simulink model "quadtank_real_manual"  (Simulink 10.0)
settings: Solver=ode45  StartTime=0.0  StopTime=inf  RelTol=1e-3  EnableMultiTasking=on
libraries: simulink x2
settings Model: Creator=kristian  LastModifiedBy=olle
settings SolverCC: ZeroCrossAlgorithm=Non-adaptive
settings DataIOCC: LimitDataPoints=on  SignalLoggingSaveFormat=ModelDataLogs
settings OptimizationCC: ExpressionDepthLimit=2147483647  InitFltsAndDblsToZero=on
settings DebuggingCC: SolverPrmCheckMsg=warning  FcnCallInpInsideContextMsg=warning  StateNameClashWarn=warning
settings SFSimCC: SimUseLocalCustomCode=on  CustomCodeUndefinedFunction=FilterOut
settings RTWCC: RTWUseLocalCustomCode=on

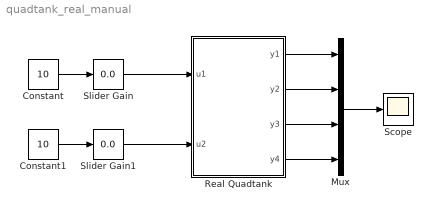
== system quadtank_real_manual ==
  Constant : Constant  Value=10
  Constant1 : Constant  Value=10
  Mux : Mux
  Real Quadtank : Subsystem  AncestorBlock=tank/Real Quadtank  VariantControl=Real  mask{h=0.05}
  Scope : Scope
  Slider Gain : simulink/Math Operations/Slider Gain  gain=0.0  low=0  high=1
  Slider Gain1 : simulink/Math Operations/Slider Gain  gain=0.0  low=0  high=1
  wires:
  Slider Gain/1 -> Real Quadtank/1(u1)
  Slider Gain1/1 -> Real Quadtank/2(u2)
  Constant/1 -> Slider Gain/1
  Constant1/1 -> Slider Gain1/1
  Mux/1 -> Scope/1
  Real Quadtank/1(y1) -> Mux/1
  Real Quadtank/2(y2) -> Mux/2
  Real Quadtank/3(y3) -> Mux/3
  Real Quadtank/4(y4) -> Mux/4

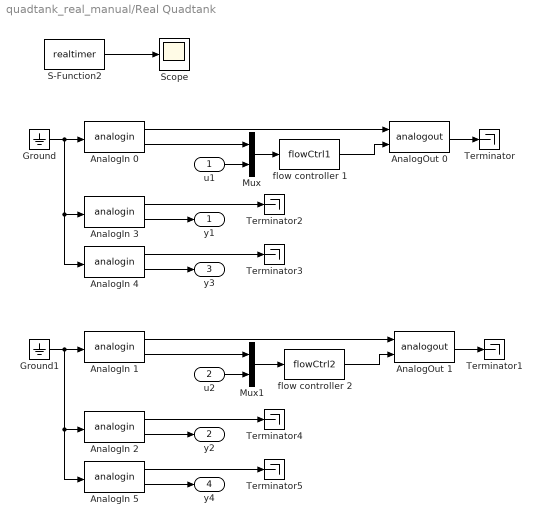
== system quadtank_real_manual/Real Quadtank ==
  u1 : Inport
  u2 : Inport  Port=2
  AnalogIn 0 : S-Function  FunctionName=analogin  Parameters=h [35]  SFunctionDeploymentMode=off  EnableBusSupport=off
  AnalogIn 1 : S-Function  FunctionName=analogin  Parameters=h [34]  SFunctionDeploymentMode=off  EnableBusSupport=off
  AnalogIn 2 : S-Function  FunctionName=analogin  Parameters=h [33]  SFunctionDeploymentMode=off  EnableBusSupport=off
  AnalogIn 3 : S-Function  FunctionName=analogin  Parameters=h [31]  SFunctionDeploymentMode=off  EnableBusSupport=off
  AnalogIn 4 : S-Function  FunctionName=analogin  Parameters=h [30]  SFunctionDeploymentMode=off  EnableBusSupport=off
  AnalogIn 5 : S-Function  FunctionName=analogin  Parameters=h [32]  SFunctionDeploymentMode=off  EnableBusSupport=off
  AnalogOut 0 : S-Function  FunctionName=analogout  Parameters=h [31]  SFunctionDeploymentMode=off  EnableBusSupport=off
  AnalogOut 1 : S-Function  FunctionName=analogout  Parameters=h [30]  SFunctionDeploymentMode=off  EnableBusSupport=off
  Ground : Ground
  Ground1 : Ground
  Mux : Mux  Inputs=2
  Mux1 : Mux  Inputs=2
  S-Function2 : S-Function  FunctionName=realtimer  Parameters=h  SFunctionDeploymentMode=off  EnableBusSupport=off
  Scope : Scope
  Terminator{,1..5} (6 alike) : Terminator
  flow controller 1 : MATLABFcn  MATLABFcn=flowCtrl1  SampleTime=0.01
  flow controller 2 : MATLABFcn  MATLABFcn=flowCtrl2  SampleTime=0.01
  y1 : Outport
  y2 : Outport  Port=2
  y3 : Outport  Port=3
  y4 : Outport  Port=4
  wires:
  AnalogIn 0/2 -> Mux/1
  AnalogIn 1/2 -> Mux1/1
  flow controller 2/1 -> AnalogOut 1/2
  Mux1/1 -> flow controller 2/1
  u2/1 -> Mux1/2
  flow controller 1/1 -> AnalogOut 0/2
  Mux/1 -> flow controller 1/1
  u1/1 -> Mux/2
  AnalogIn 5/1 -> Terminator5/1
  AnalogIn 2/1 -> Terminator4/1
  Ground1/1 -> AnalogIn 1/1, AnalogIn 2/1, AnalogIn 5/1
  AnalogIn 5/2 -> y4/1
  AnalogIn 2/2 -> y2/1
  AnalogIn 4/1 -> Terminator3/1
  AnalogIn 3/1 -> Terminator2/1
  Ground/1 -> AnalogIn 4/1, AnalogIn 3/1, AnalogIn 0/1
  AnalogIn 4/2 -> y3/1
  AnalogIn 3/2 -> y1/1
  AnalogOut 1/1 -> Terminator1/1
  AnalogIn 1/1 -> AnalogOut 1/1
  AnalogOut 0/1 -> Terminator/1
  AnalogIn 0/1 -> AnalogOut 0/1
  S-Function2/1 -> Scope/1
